simulink model "v10_onebit_compare"  (R2019b)
settings: Solver=VariableStepAuto  StartTime=0.0  StopTime=inf  RelTol=1e-3
settings Model: Creator=MARAT  LastModifiedBy=Marat
settings SFSimCC: CustomCodeUndefinedFunction=UseInterfaceOnly

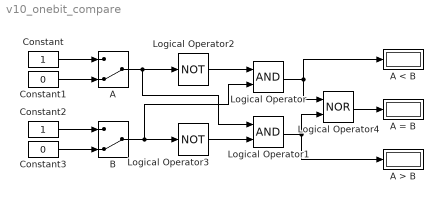
== system v10_onebit_compare ==
  A : ManualSwitch  CurrentSetting=0
  A < B : Display
  A = B : Display
  A > B : Display
  B : ManualSwitch  CurrentSetting=0
  Constant : Constant  OutDataTypeStr=boolean
  Constant1 : Constant  Value=0  OutDataTypeStr=boolean
  Constant2 : Constant  OutDataTypeStr=boolean
  Constant3 : Constant  Value=0  OutDataTypeStr=boolean
  Logical Operator : Logic  AllPortsSameDT=off  OutDataTypeStr=boolean
  Logical Operator1 : Logic  AllPortsSameDT=off  OutDataTypeStr=boolean
  Logical Operator2 : Logic  Operator=NOT  AllPortsSameDT=off  OutDataTypeStr=boolean
  Logical Operator3 : Logic  Operator=NOT  AllPortsSameDT=off  OutDataTypeStr=boolean
  Logical Operator4 : Logic  Operator=NOR  AllPortsSameDT=off  OutDataTypeStr=boolean
  wires:
  Constant1/1 -> A/2
  Constant/1 -> A/1
  Constant2/1 -> B/1
  Constant3/1 -> B/2
  A/1 -> Logical Operator1/1, Logical Operator2/1
  B/1 -> Logical Operator/2, Logical Operator3/1
  Logical Operator2/1 -> Logical Operator/1
  Logical Operator3/1 -> Logical Operator1/2
  Logical Operator/1 -> A < B/1, Logical Operator4/1
  Logical Operator1/1 -> Logical Operator4/2, A > B/1
  Logical Operator4/1 -> A = B/1
